simulink model "YixuanMeng_SL_CT"  (R2019b)
settings: Solver=FixedStepDiscrete  StartTime=0.0  StopTime=6000  FixedStep=1  RelTol=1e-3  EnableMultiTasking=on
settings Model: SnapshotBufferSize=100  SnapshotInterval=1  Creator=dell  LastModifiedBy=DELL-PC
settings SolverCC: AutoInsertRateTranBlk=on
settings DataIOCC: LimitDataPoints=on  ReturnWorkspaceOutputs=off
settings OptimizationCC: LifeSpan=inf
settings DebuggingCC: AllowSymbolicDim=off  SFUnexpectedBacktrackingDiag=warning  SFNoUnconditionalDefaultTransitionDiag=warning  SFExecutionAtInitializationDiag=none  ArithmeticOperatorsInVariantConditions=warning
settings SFSimCC: SimUseLocalCustomCode=off  CustomCodeUndefinedFunction=UseInterfaceOnly
settings RTWCC: RTWUseLocalCustomCode=off
settings CodeAppCC: StateflowObjectComments=on
settings GRTTargetCC: TargetLangStandard=C89/C90 (ANSI)
settings ConfigComp: CovMetricSettings=dw  CovHtmlReporting=on  CovSaveCumulativeToWorkspaceVar=on  CovSaveSingleToWorkspaceVar=on  CovShowResultsExplorer=off  CovExternalEMLEnable=off

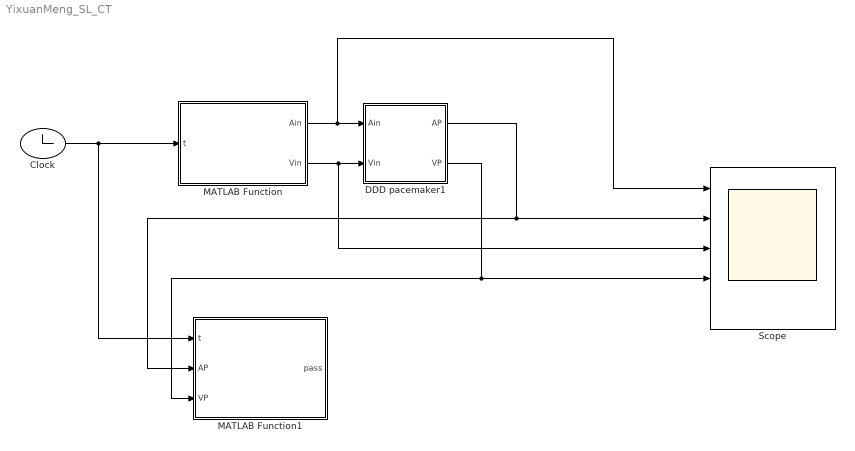
== system YixuanMeng_SL_CT ==
  Clock : Clock
  DDD pacemaker1 : Subsystem
  MATLAB Function : MATLAB Function  TreatAsAtomicUnit=on
  MATLAB Function1 : MATLAB Function  TreatAsAtomicUnit=on
  Scope : Scope  NumInputPorts=5
  wires:
  DDD pacemaker1/2(VP) -> Scope/4, MATLAB Function1/3(VP)
  MATLAB Function/2(Vin) -> DDD pacemaker1/2(Vin), Scope/3
  DDD pacemaker1/1(AP) -> Scope/2, MATLAB Function1/2(AP)
  MATLAB Function/1(Ain) -> DDD pacemaker1/1(Ain), Scope/1
  Clock/1 -> MATLAB Function1/1(t), MATLAB Function/1(t)

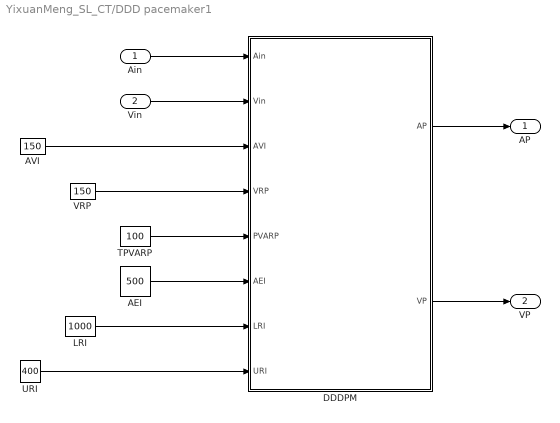
== system YixuanMeng_SL_CT/DDD pacemaker1 ==
  Ain : Inport
  Vin : Inport  Port=2
  AEI : Constant  Value=500
  AVI : Constant  Value=150  OutDataTypeStr=uint16
  DDDPM : Stateflow chart  TreatAsAtomicUnit=on
  LRI : Constant  Value=1000  OutDataTypeStr=uint16
  TPVARP : Constant  Value=100  OutDataTypeStr=uint16
  URI : Constant  Value=400  OutDataTypeStr=uint16
  VRP : Constant  Value=150  OutDataTypeStr=uint16
  AP : Outport
  VP : Outport  Port=2
  wires:
  DDDPM/2(VP) -> VP/1
  DDDPM/1(AP) -> AP/1
  Vin/1 -> DDDPM/2(Vin)
  Ain/1 -> DDDPM/1(Ain)
  AVI/1 -> DDDPM/3(AVI)
  VRP/1 -> DDDPM/4(VRP)
  TPVARP/1 -> DDDPM/5(PVARP)
  URI/1 -> DDDPM/8(URI)
  LRI/1 -> DDDPM/7(LRI)
  AEI/1 -> DDDPM/6(AEI)

== stateflow chart YixuanMeng_SL_CT/DDD pacemaker1/DDDPM ==
  settings: updateMethod=DISCRETE  sampleTime=1
  state DDDPM
    state AVI [parallel]
      settings: executionOrder=3
      state ActiveAVI
      state CAVI
      state IdleAVI
      (default) -> IdleAVI : {VP=false,VP1=false;}
      ActiveAVI -> ActiveAVI [order 3] : [tmpAVI>0]/{tmpAVI=tmpAVI-1;}
      IdleAVI -> ActiveAVI : [AS==true || AP1==true]/
          | {tmpAVI=AVI;}
      ActiveAVI -> CAVI [order 1] : [tmpAVI<=0&&enterURI==true]/
          | {VP=true, VP1=true;}
      ActiveAVI -> IdleAVI [order 2] : [VS==true || VP1==true]
      CAVI -> IdleAVI : {VP=false,VP1=false;}
    state URI [parallel]
      settings: executionOrder=1
      state IdleURI
      state ActiveURI
      (default) -> IdleURI : {enterURI=true;}
      IdleURI -> ActiveURI : [VP1==true || VS==true]/
          | {tmpURI=URI, enterURI=false;}
      ActiveURI -> IdleURI [order 3] : [tmpURI<=0]/{enterURI=true;}
      ActiveURI -> ActiveURI [order 2] : [tmpURI>0]/{tmpURI = tmpURI - 1;}
      ActiveURI -> ActiveURI [order 1] : [VS==true || VP1==true]/
          | {tmpURI=URI, enterURI=false;}
    state PVARP [parallel]
      settings: executionOrder=5
      state AinPVARP
      state IdlePVARP
      state ActivePVARP
      state PVARPAR
      IdlePVARP -> AinPVARP [order 1] : [Ain==true]/{AS=true}
      AinPVARP -> IdlePVARP : {AS=false;}
      (default) -> IdlePVARP : {AS=false;}
      IdlePVARP -> ActivePVARP [order 2] : [VS==true || VP1==true]/{tmpPVARP=PVARP;}
      ActivePVARP -> IdlePVARP [order 3] : [tmpPVARP<=0]
      ActivePVARP -> ActivePVARP [order 2] : [tmpPVARP>0]/
          | {tmpPVARP = tmpPVARP - 1;}
      PVARPAR -> ActivePVARP : {AR=false,tmpPVARP = tmpPVARP - 1;}
      ActivePVARP -> PVARPAR [order 1] : [Ain==true]/{AR=true;}
    state LRI [parallel]
      settings: executionOrder=2
      state IdleLRI
      state LRIVP
      state ActiveLRI
      IdleLRI -> IdleLRI [order 1] : [VS==true||VP1==true]/
          | {tmpLRI=LRI;}
      (default) -> IdleLRI : {tmpLRI = LRI,APLRI=2,AP=false,AP1=false;}
      IdleLRI -> IdleLRI [order 3] : [tmpLRI>AVI]/
          | {tmpLRI = tmpLRI-1;}
      LRIVP -> IdleLRI : /{VP=false, VP1=false, tmpLRI=LRI;}
      IdleLRI -> ActiveLRI [order 4] : [tmpLRI<=AVI]/
          | {AP=true,APLRI=1,AP1=true,tmpLRI=tmpLRI-1;}
      IdleLRI -> ActiveLRI [order 2] : [AS==true]/{tmpLRI=tmpLRI-1;}
      ActiveLRI -> IdleLRI [order 2] : [VS==true || VP1==true]/{tmpLRI=LRI;}
      ActiveLRI -> LRIVP [order 4] : [tmpLRI<=0]/
          | {VP=true,VP1=true;}
      ActiveLRI -> ActiveLRI [order 3] : [tmpLRI>0]
          | /{tmpLRI=tmpLRI-1;}
      ActiveLRI -> ActiveLRI [order 1] : [APLRI==1]/
          | {APLRI=APLRI+1,AP=false,AP1=false,
          | tmpLRI=tmpLRI-1;}
    state VRP [parallel]
      settings: executionOrder=4
      state VRPVS
      state IdleVRP
      state ActiveVRP
      IdleVRP -> VRPVS [order 1] : [Vin==true]/{VS=true}
      VRPVS -> ActiveVRP : {tmpVRP=VRP,VS=false;}
      (default) -> IdleVRP : {VS=false}
      IdleVRP -> ActiveVRP [order 2] : [VP1==true]/{tmpVRP=VRP;}
      ActiveVRP -> ActiveVRP [order 1] : [tmpVRP>0]/{tmpVRP= tmpVRP - 1;}
      ActiveVRP -> IdleVRP [order 2] : [tmpVRP<=0]
  (default) -> DDDPM : {VS=false, VP1=false, VP=false, AS=false,AR=false,AP1=false,  APLRI=2,  AP=false,  enterURI=true, tmpVRP=VRP, tmpPVARP = PVARP, tmpAVI= AVI, tmpLRI = LRI, tmpURI = URI;}
  data: Ain input; VS local; Vin input; AP output; VP output; tmpVRP local; AS local; tmpPVARP local; tmpAVI local; enterURI local; tmpLRI local; tmpURI local; APLRI local; VP1 local; AP1 local; AR local; AVI input uint16; VRP input uint16 =150; PVARP input uint16; AEI input; LRI input uint16; URI input uint16; APLRI1 local

== matlab function YixuanMeng_SL_CT/MATLAB Function ==
  data: t input; Ain output; Vin output
function [Ain,Vin] = PM_tester_in(t)

%Ain
%if mod(t-50,200)==0
if t==199 || t==1204
    Ain=true;
else
    Ain=false;
end




%Vin
%if mod(t-150,200)==0
if t==1202
    Vin=true;
else
    Vin=false;
end

Vin=false;

== matlab function YixuanMeng_SL_CT/MATLAB Function1 ==
  data: t input; pass output; AP input; VP input
function pass = PM_tester_out(t,AP,VP)
pass=true;
% Evaluating PM outputs
% if t==200
%     if AS==true
%         
%     else
%         pass=false;
%         return;
%     end
% end

if t==350
    if VP==true
        
    else
        pass=false;
        return;
    end
end

if t==1201
    if AP==true
        
    else
        pass=false;
        return;
    end
end

% if t==1203
%     if VS==true
%         
%     else
%         pass=false;
%         return;
%     end
% end

% if t==1205
%     if AR==true
%         
%     else
%         pass=false;
%         return;
%     end
% end
if pass==false
    pass
end
